simulink model "simple_relay_plant"  (R2015a)
settings: Solver=ode45  StartTime=0.0  StopTime=tmax  RelTol=1e-3
values from neighbouring files (symbols this model uses):
  b = 1    [testing_relay_plant_positive_feedback.m]
  d = 1    [testing_relay_plant_positive_feedback.m]
settings Model: Creator=ra428  LastModifiedBy=ra428

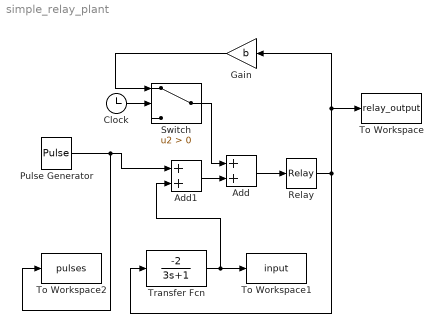
== system simple_relay_plant ==
  Add : Sum
  Add1 : Sum
  Clock : Clock
  Gain : Gain  Gain=b
  Pulse Generator : DiscretePulseGenerator  PulseType=Time based  Period=80  PulseWidth=50  PhaseDelay=30
  Relay : Relay  OnSwitchValue=0  OffSwitchValue=0  OnOutputValue=d  OffOutputValue=-d
  Switch : Switch  Criteria=u2 > Threshold
  To Workspace : ToWorkspace  VariableName=relay_output  SaveFormat=Timeseries  SampleTime=-1
  To Workspace1 : ToWorkspace  VariableName=input  SaveFormat=Timeseries  SampleTime=-1
  To Workspace2 : ToWorkspace  VariableName=pulses  SaveFormat=Timeseries  SampleTime=-1
  Transfer Fcn : TransferFcn  Numerator=[-2]  Denominator=[3 1]
  wires:
  Relay/1 -> To Workspace/1, Gain/1, Transfer Fcn/1
  Add/1 -> Relay/1
  Gain/1 -> Switch/1
  Transfer Fcn/1 -> Add1/2, To Workspace1/1
  Switch/1 -> Add/1
  Clock/1 -> Switch/2
  Pulse Generator/1 -> To Workspace2/1, Add1/1
  Add1/1 -> Add/2
